simulink model "guid_full_loop"  (R2021a)
settings: Solver=VariableStepAuto  StartTime=0.0  StopTime=5  RelTol=1e-3
values from neighbouring files (symbols this model uses):
  Ahg3 = blkdiag(Ahg3, Ahcg)    [ranger_full_indi_sim.m]
  Bhg3 = blkdiag(Bhg3, Bhcg)    [ranger_full_indi_sim.m]
  Chg3 = blkdiag(Chg3, Chcg)    [ranger_full_indi_sim.m]
  Dhg3 = blkdiag(Dhg3, Dhcg)    [ranger_full_indi_sim.m]
  Kdg = [2.0; 2.0; 1.8]    [ranger_full_indi_sim.m]
  Kpg = [0.581; 0.581; 0.5943]    [ranger_full_indi_sim.m]
settings Model: Creator=AutomZ2-RG02B04  LastModifiedBy=AutomZ2-RG02A02
settings SolverCC: AlgebraicLoopSolver=TrustRegion

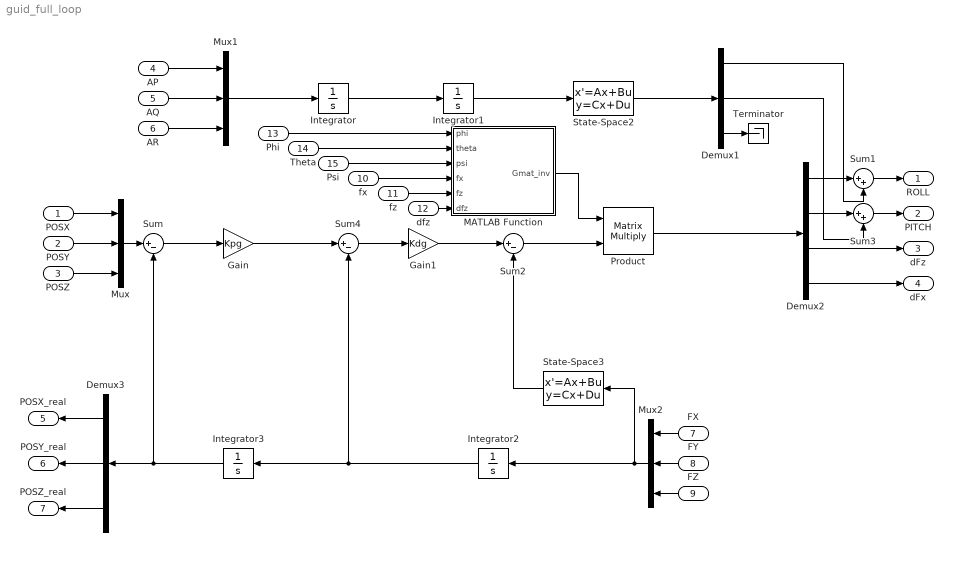
== system guid_full_loop ==
  POSX : Inport
  POSY : Inport  Port=2
  POSZ : Inport  Port=3
  AP : Inport  Port=4
  AQ : Inport  Port=5
  AR : Inport  Port=6
  FX : Inport  Port=7
  FY : Inport  Port=8
  FZ : Inport  Port=9
  fx : Inport  Port=10
  fz : Inport  Port=11
  dfz : Inport  Port=12
  Phi : Inport  Port=13
  Theta : Inport  Port=14
  Psi : Inport  Port=15
  Demux1 : Demux  Outputs=3
  Demux2 : Demux
  Demux3 : Demux  Outputs=3
  Gain : Gain  Gain=Kpg
  Gain1 : Gain  Gain=Kdg
  Integrator{,1..3} (4 alike) : Integrator
  MATLAB Function : MATLAB Function  TreatAsAtomicUnit=on
  Mux : Mux  Inputs=3
  Mux1 : Mux  Inputs=3
  Mux2 : Mux  Inputs=3
  Product : Product  Multiplication=Matrix(*)
  State-Space2 : StateSpace  A=Ahg3  B=Bhg3  C=Chg3  D=Dhg3  InitialCondition=0
  State-Space3 : StateSpace  A=Ahg3  B=Bhg3  C=Chg3  D=Dhg3  InitialCondition=0
  Sum : Sum  Inputs=|+-
  Sum1 : Sum  Inputs=|++
  Sum2 : Sum  Inputs=|+-
  Sum3 : Sum  Inputs=|++
  Sum4 : Sum  Inputs=|+-
  Terminator : Terminator
  ROLL : Outport
  PITCH : Outport  Port=2
  dFz : Outport  Port=3
  dFx : Outport  Port=4
  POSX_real : Outport  Port=5
  POSY_real : Outport  Port=6
  POSZ_real : Outport  Port=7
  wires:
  Sum/1 -> Gain/1
  POSY/1 -> Mux/2
  POSZ/1 -> Mux/3
  Mux/1 -> Sum/1
  POSX/1 -> Mux/1
  Gain/1 -> Sum4/1
  Sum4/1 -> Gain1/1
  Gain1/1 -> Sum2/1
  AP/1 -> Mux1/1
  AQ/1 -> Mux1/2
  AR/1 -> Mux1/3
  Mux1/1 -> Integrator/1
  Mux2/1 -> Integrator2/1, State-Space3/1
  Integrator/1 -> Integrator1/1
  Integrator1/1 -> State-Space2/1
  State-Space2/1 -> Demux1/1
  Demux1/3 -> Terminator/1
  FX/1 -> Mux2/1
  FY/1 -> Mux2/2
  Integrator2/1 -> Sum4/2, Integrator3/1
  Integrator3/1 -> Demux3/1, Sum/2
  FZ/1 -> Mux2/3
  State-Space3/1 -> Sum2/2
  Demux2/3 -> dFz/1
  Sum2/1 -> Product/2
  Product/1 -> Demux2/1
  Demux2/4 -> dFx/1
  Demux2/1 -> Sum1/1
  Sum1/1 -> ROLL/1
  Demux1/1 -> Sum1/2
  Demux2/2 -> Sum3/1
  Demux1/2 -> Sum3/2
  Sum3/1 -> PITCH/1
  MATLAB Function/1(Gmat_inv) -> Product/1
  fx/1 -> MATLAB Function/4(fx)
  fz/1 -> MATLAB Function/5(fz)
  dfz/1 -> MATLAB Function/6(dfz)
  Phi/1 -> MATLAB Function/1(phi)
  Theta/1 -> MATLAB Function/2(theta)
  Psi/1 -> MATLAB Function/3(psi)
  Demux3/1 -> POSX_real/1
  Demux3/3 -> POSZ_real/1
  Demux3/2 -> POSY_real/1

== matlab function guid_full_loop/MATLAB Function ==
  data: phi input; Gmat_inv output; theta input; psi input; fx input; fz input; dfz input
function Gmat_inv = computeGmat_inv(phi, theta, psi, fx, fz, dfz)

gi_pitch_eff_scaling = 1.0;
gi_lift_eff_scaling = 1.0;
gi_thrust_eff_scaling = 1.0;

sphi = sin(phi); cphi = cos(phi);
stheta = sin(theta); ctheta = cos(theta);
spsi = sin(psi); cpsi = cos(psi);

Gmat = zeros(3,4);

% dPhi (Roll)
Gmat(1,1) = fx * (-spsi * cphi * stheta) + fz * (spsi * cphi * ctheta);
Gmat(2,1) = fx * (cpsi * cphi * stheta) + fz * (-cpsi * cphi * ctheta);
Gmat(3,1) = fx * (sphi * stheta) + fz * (-sphi * ctheta);

% dTheta (Pitch)
Gmat(1,2) = fx * (-cpsi * stheta - spsi * sphi * ctheta) + ...
            fz * (cpsi * ctheta - spsi * sphi * stheta) * gi_pitch_eff_scaling + ...
            (cpsi * stheta + spsi * sphi * ctheta) * dfz;

Gmat(2,2) = fx * (-spsi * stheta + cpsi * sphi * ctheta) + ...
            fz * (spsi * ctheta + cpsi * sphi * stheta) * gi_pitch_eff_scaling + ...
            (spsi * stheta - cpsi * sphi * ctheta) * dfz;

Gmat(3,2) = fx * (-cphi * ctheta) + ...
            fz * (-cphi * stheta) * gi_pitch_eff_scaling + ...
            cphi * ctheta * dfz;

% dfz
Gmat(1,3) = (cpsi * stheta + spsi * sphi * ctheta) * gi_lift_eff_scaling;
Gmat(2,3) = (spsi * stheta - cpsi * sphi * ctheta) * gi_lift_eff_scaling;
Gmat(3,3) = cphi * ctheta * gi_lift_eff_scaling;

% dfx
Gmat(1,4) = (cpsi * ctheta - spsi * sphi * stheta) * gi_thrust_eff_scaling;
Gmat(2,4) = (spsi * ctheta + cpsi * sphi * stheta) * gi_thrust_eff_scaling;
Gmat(3,4) = -stheta * cphi * gi_thrust_eff_scaling;

Gmat_inv = pinv(Gmat);

end
